simulink model "motor_modeling_final"  (R2021a)
settings: Solver=VariableStepAuto  StartTime=0.0  StopTime=10.0  RelTol=1e-3
undefined symbols (not defined in the file): b, J, Ld, Lq, P, PM, Pm, Rs, TL
settings Model: Creator=dell  LastModifiedBy=dell

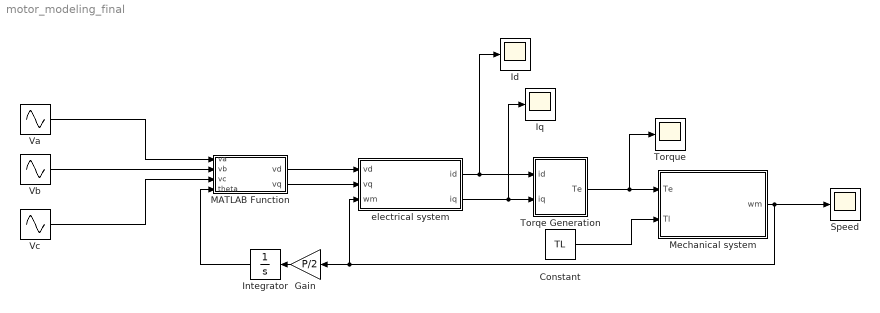
== system motor_modeling_final ==
  Constant : Constant  Value=TL
  Gain : Gain  Gain=P/2
  Id : Scope
  Integrator : Integrator
  Iq : Scope
  MATLAB Function : MATLAB Function  TreatAsAtomicUnit=on
  Mechanical system : Subsystem
  Speed : Scope
  Torqe Generation : Subsystem
  Torque : Scope
  Va : Sin  Amplitude=220  Frequency=2*pi*60  SampleTime=0
  Vb : Sin  Amplitude=220  Frequency=2*pi*60  Phase=-2*pi/3  SampleTime=0
  Vc : Sin  Amplitude=220  Frequency=2*pi*60  Phase=2*pi/3  SampleTime=0
  electrical system : Subsystem
  wires:
  electrical system/1(id) -> Id/1, Torqe Generation/1(id)
  Constant/1 -> Mechanical system/2(Tl)
  Mechanical system/1(wm) -> Speed/1, Gain/1, electrical system/3(wm)
  electrical system/2(iq) -> Iq/1, Torqe Generation/2("iq ")
  Torqe Generation/1(Te) -> Torque/1, Mechanical system/1(Te)
  Gain/1 -> Integrator/1
  MATLAB Function/2(vq) -> electrical system/2(vq)
  MATLAB Function/1(vd) -> electrical system/1(vd)
  Integrator/1 -> MATLAB Function/4(theta)
  Vb/1 -> MATLAB Function/2(vb)
  Vc/1 -> MATLAB Function/3(vc)
  Va/1 -> MATLAB Function/1(va)

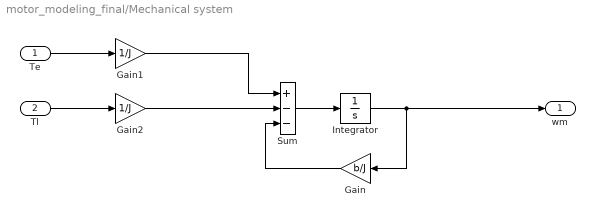
== system motor_modeling_final/Mechanical system ==
  Te : Inport
  Tl : Inport  Port=2
  Gain : Gain  Gain=b/J
  Gain1 : Gain  Gain=1/J
  Gain2 : Gain  Gain=1/J
  Integrator : Integrator
  Sum : Sum  Inputs=+--
  wm : Outport  VectorParamsAs1DForOutWhenUnconnected=off
  wires:
  Integrator/1 -> wm/1, Gain/1
  Gain1/1 -> Sum/1
  Gain2/1 -> Sum/2
  Sum/1 -> Integrator/1
  Gain/1 -> Sum/3
  Te/1 -> Gain1/1
  Tl/1 -> Gain2/1

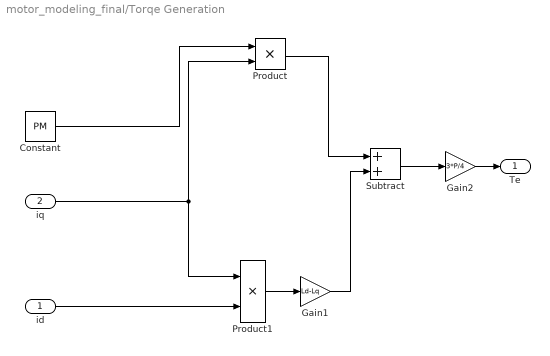
== system motor_modeling_final/Torqe Generation ==
  id : Inport
  "iq " : Inport  Port=2
  Constant : Constant  Value=PM
  Gain1 : Gain  Gain=Ld-Lq
  Gain2 : Gain  Gain=3*P/4
  Product : Product
  Product1 : Product
  Subtract : Sum
  Te : Outport  VectorParamsAs1DForOutWhenUnconnected=off
  wires:
  id/1 -> Product1/2
  Constant/1 -> Product/1
  "iq "/1 -> Product1/1, Product/2
  Product/1 -> Subtract/1
  Subtract/1 -> Gain2/1
  Gain2/1 -> Te/1
  Product1/1 -> Gain1/1
  Gain1/1 -> Subtract/2

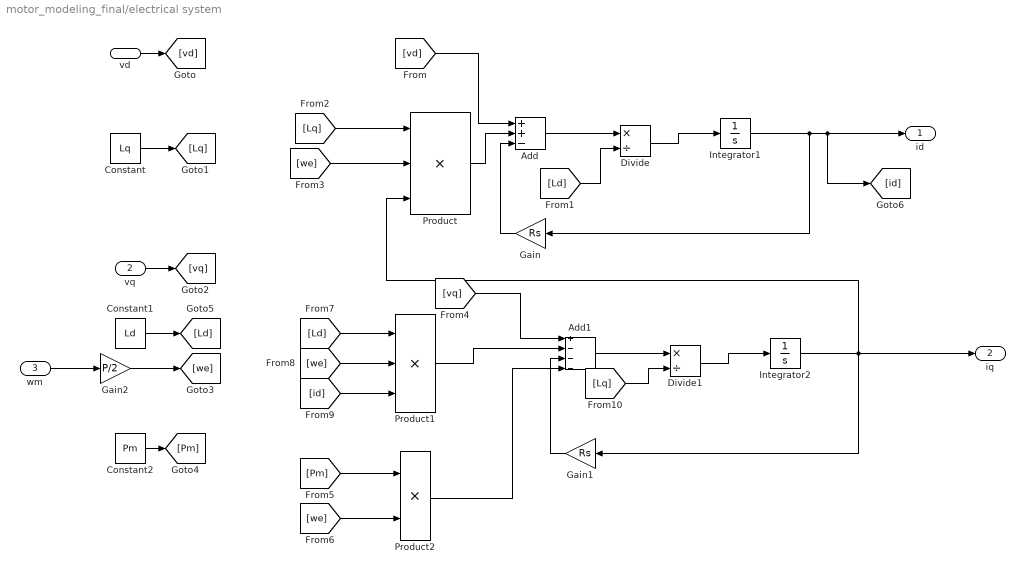
== system motor_modeling_final/electrical system ==
  vd : Inport
  vq : Inport  Port=2
  wm : Inport  Port=3
  Add : Sum  Inputs=++-
  Add1 : Sum  Inputs=+---
  Constant : Constant  Value=Lq
  Constant1 : Constant  Value=Ld
  Constant2 : Constant  Value=Pm
  Divide : Product  Inputs=*/
  Divide1 : Product  Inputs=*/
  Gain : Gain  Gain=Rs
  Gain1 : Gain  Gain=Rs
  Gain2 : Gain  Gain=P/2
  Integrator1 : Integrator
  Integrator2 : Integrator
  Product : Product  Inputs=3
  Product1 : Product  Inputs=3
  Product2 : Product
  id : Outport
  iq : Outport  Port=2
  wires:
  Product/1 -> Add/2
  Gain/1 -> Add/3
  Integrator1/1 -> Gain/1, [id], id/1
  Add/1 -> Divide/1
  Divide/1 -> Integrator1/1
  Divide1/1 -> Integrator2/1
  Add1/1 -> Divide1/1
  Gain1/1 -> Add1/3
  Integrator2/1 -> Product/3, iq/1, Gain1/1
  vd/1 -> [vd]
  Constant1/1 -> [Ld]
  Constant/1 -> [Lq]
  Constant2/1 -> [Pm]
  wm/1 -> Gain2/1
  vq/1 -> [vq]
  [vd] -> Add/1
  [Ld] -> Divide/2
  [Lq] -> Product/1
  [we] -> Product/2
  [vq] -> Add1/1
  Product1/1 -> Add1/2
  Product2/1 -> Add1/4
  [Pm] -> Product2/1
  [we] -> Product2/2
  [Ld] -> Product1/1
  [we] -> Product1/2
  [id] -> Product1/3
  [Lq] -> Divide1/2
  Gain2/1 -> [we]

== matlab function motor_modeling_final/MATLAB Function ==
  data: va input; vd output; vb input; vc input; theta input; vq output
function [vd,vq] = fcn(va,vb,vc,theta)
vd=(2/3)*(va*cos(theta)+vb*cos(theta-(2*pi/3))+vc*cos(theta+(2*pi/3)));
vq=(2/3)*(-va*sin(theta)-vb*sin(theta-(2*pi/3))-vc*sin(theta+(2*pi/3)));
end
